simulink model "testmdl"  (R2023b)
settings: Solver=FixedStepAuto  StartTime=0.0  StopTime=ts  FixedStep=1e-3  RelTol=1e-3
undefined symbols (not defined in the file or in its folder): c, f
settings Model: Creator=LEONELLIF  LastModifiedBy=LEONELLIF

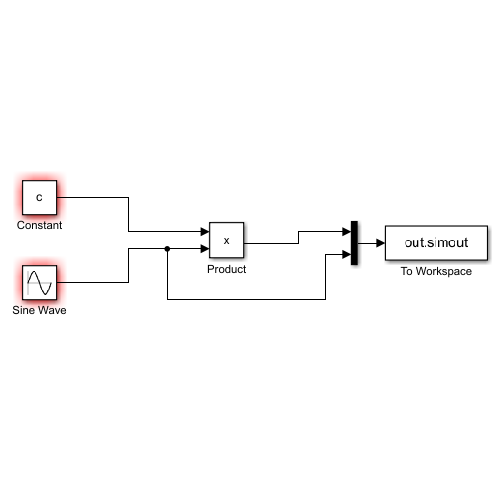
[thumbnail: Simulink's stored preview of the top-level diagram]
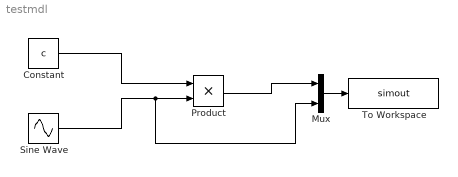
== system testmdl ==
  Constant : Constant  Value=c
  Mux : Mux  Inputs=2
  Product : Product
  Sine Wave : Sin  Frequency=f  SampleTime=0
  To Workspace : ToWorkspace  VariableName=simout  SaveFormat=Timeseries  SampleTime=-1
  wires:
  Constant/1 -> Product/1
  Sine Wave/1 -> Mux/2, Product/2
  Product/1 -> Mux/1
  Mux/1 -> To Workspace/1
